simulink model "IndicatorControl"  (R2025a)
settings: Solver=FixedStepDiscrete  StartTime=0.0  StopTime=10.0  FixedStep=0.1  RelTol=1e-3
settings Model: Creator=amirperreh  LastModifiedBy=amirperreh
settings OptimizationCC: DefaultParameterBehavior=Inlined  EnhancedBackFolding=on  PassReuseOutputArgsAs=Individual arguments  OptimizeBlockOrder=speed  DifferentSizesBufferReuse=on  OptimizationCustomize=off  EfficientTunableParamExpr=on
settings DebuggingCC: ParameterTunabilityLossMsg=error
settings HardwareCC: ProdBitPerPointer=32.0  ProdBitPerSizeT=32.0  ProdBitPerPtrDiffT=32.0  ProdLargestAtomicInteger=Long  ProdLargestAtomicFloat=Double  ProdWordSize=32.0  ProdHWDeviceType=ARM Compatible->ARM Cortex-M
settings SFSimCC: MATLABDynamicMemAlloc=off
settings RTWCC: SystemTargetFile=ert.tlc  GenCodeOnly=on  TemplateMakefile=ert_default_tmf  Description=Embedded Coder
settings CodeAppCC: ForceParamTrailComments=on  IgnoreCustomStorageClasses=off  OperatorAnnotations=on  SimulinkDataObjDesc=on  SFDataObjDesc=on  InsertBlockDesc=on
settings ERTTargetCC: ExtModeTransport=0.0  ExtModeStaticAlloc=off  ExtModeMexFile=ext_comm  ExtModeIntrfLevel=Level1  ERTCustomFileTemplate=example_file_process.tlc  UtilityFuncGeneration=Shared location  GenerateSampleERTMain=on  CodeInterfacePackaging=Reusable function

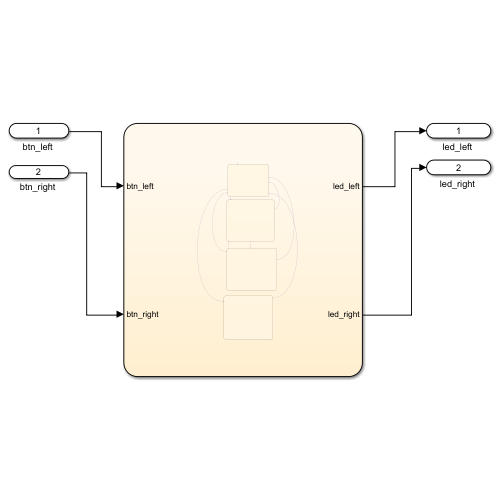
[thumbnail: Simulink's stored preview of the top-level diagram]
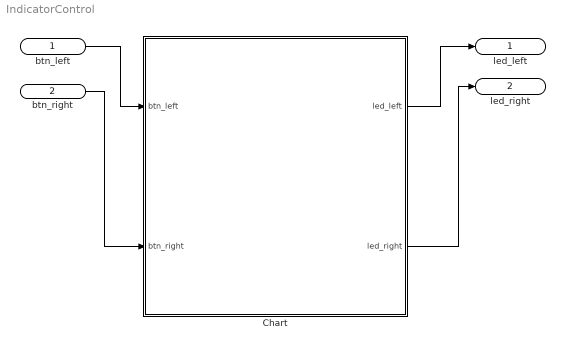
== system IndicatorControl ==
  "btn_left " : Inport
  "btn_right " : Inport  Port=2
  Chart : Stateflow chart  TreatAsAtomicUnit=on
  "led_left " : Outport
  "led_right " : Outport  Port=2
  wires:
  "btn_right "/1 -> Chart/2(btn_right)
  "btn_left "/1 -> Chart/1(btn_left)
  Chart/1(led_left) -> "led_left "/1
  Chart/2(led_right) -> "led_right "/1

== stateflow chart IndicatorControl/Chart ==
  settings: executeAtInitialization=1
  state OFF
    entry:
    led_left = false;
    led_right = false;
    hold_counter_L = 0;
    hold_counter_R = 0;
    blink_counter = 0;
    blink_state = false;
    during:
    if btn_left
    hold_counter_L = hold_counter_L + 1;
    else
    hold_counter_L = 0;
    end
    if btn_right
    hold_counter_R = hold_counter_R + 1;
    else
    hold_counter_R = 0;
    end
  state LEFT_ON
    entry:
    blink_counter = 0;
    blink_state = true;
    hold_counter_L = 0;
    hold_counter_R = 0;
    during:
    blink_counter = blink_counter + 1;
    if blink_counter >= 3
    blink_counter = 0;
    end
    if blink_counter == 0
    blink_state = ~blink_state;
    end
    led_left = blink_state;
    led_right = false;
    if btn_left
    hold_counter_L = hold_counter_L + 1;
    else
    hold_counter_L = 0;
    end
    if btn_right
    hold_counter_R = hold_counter_R + 1;
    else
    hold_counter_R = 0;
    end
  state RIGHT_ON
    entry:
    blink_counter = 0;
    blink_state = true;
    hold_counter_L = 0;
    hold_counter_R = 0;
    during:
    blink_counter = blink_counter + 1;
    if blink_counter >= 3
    blink_counter = 0;
    end
    if blink_counter == 0
    blink_state = ~blink_state;
    end
    led_left = false;
    led_right = blink_state;
    if btn_left
    hold_counter_L = hold_counter_L + 1;
    else
    hold_counter_L = 0;
    end
    if btn_right
    hold_counter_R = hold_counter_R + 1;
    else
    hold_counter_R = 0;
    end
  state HAZARD
    entry:
    blink_counter = 0;
    blink_state = true;
    hold_counter_L = 0;
    hold_counter_R = 0;
    during:
    blink_counter = blink_counter + 1;
    if blink_counter >= 3
    blink_counter = 0;
    end
    if blink_counter == 0
    blink_state = ~blink_state;
    end
    led_left = blink_state;
    led_right = blink_state;
    if btn_left
    hold_counter_L = hold_counter_L + 1;
    else
    hold_counter_L = 0;
    end
    if btn_right
    hold_counter_R = hold_counter_R + 1;
    else
    hold_counter_R = 0;
    end
  (default) -> OFF
  RIGHT_ON -> OFF [order 2] : [~btn_right && hold_counter_R >= 10]
  LEFT_ON -> OFF [order 2] : [~btn_left && hold_counter_L >= 10]
  OFF -> HAZARD [order 3] : [btn_left && btn_right && hold_counter_L >= 10 && hold_counter_R >= 10]
  OFF -> RIGHT_ON [order 2] : [btn_right && ~btn_left && hold_counter_R >= 10]
  HAZARD -> OFF : [(btn_left || btn_right) && (hold_counter_L >= 10 || hold_counter_R >= 10)]
  OFF -> LEFT_ON [order 1] : [btn_left && ~btn_right && hold_counter_L >= 10]
  RIGHT_ON -> LEFT_ON [order 1] : [btn_left && hold_counter_L >= 10]
  LEFT_ON -> RIGHT_ON [order 1] : [btn_right && hold_counter_R >= 10]
  data: btn_left input boolean; btn_right input boolean; led_left output boolean; led_right output boolean; blink_counter local uint8; blink_state local boolean; hold_counter_L local uint8; hold_counter_R local uint8
